simulink model "no_signal"  (R2017a)
settings: Solver=VariableStepAuto  StartTime=0.0  StopTime=10.0  RelTol=1e-3
settings Model: Creator=joaomanito  LastModifiedBy=joaomanito

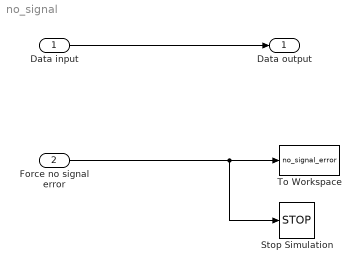
== system no_signal ==
  Data input : Inport
  Force no signal error : Inport  Port=2
  Stop Simulation : Stop
  To Workspace : ToWorkspace  VariableName=no_signal_error  SaveFormat=Timeseries  SampleTime=-1
  Data output : Outport
  wires:
  Data input/1 -> Data output/1
  Force no signal error/1 -> Stop Simulation/1, To Workspace/1
